simulink model "Platoon"  (Simulink 8.8)
settings: Solver=ode45  StartTime=0  StopTime=120  RelTol=1e-3  EnableMultiTasking=on
libraries: Solver_SF x5
settings Model: Creator=dhall  LastModifiedBy=mkhan  ExtModeTrigMode=oneshot  ExtModeArmWhenConnect=off
settings DataIOCC: LimitDataPoints=off  SignalLoggingName=sigsOut
settings OptimizationCC: BooleanDataType=off  LocalBlockOutputs=off  InitFltsAndDblsToZero=on
settings DebuggingCC: SaveWithParameterizedLinksMsg=none  SignalResolutionControl=TryResolveAllWithWarning  MultiTaskDSMMsg=warning  MultiTaskCondExecSysMsg=none  SFExecutionAtInitializationDiag=warning
settings HardwareCC: TargetUnknown=on
settings GRTTargetCC: TargetFcnLib=ansi_tfl_tmw.mat  CompOptLevelCompliant=off
settings ConfigComp: CovSFcnEnable=off

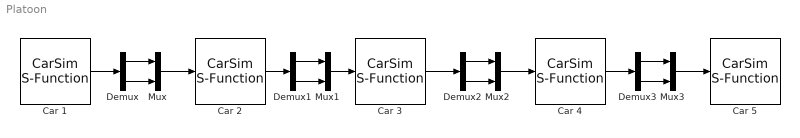
== system Platoon ==
  Car 1 : Solver_SF/CarSim S-Function  Priority=1  SIMFILE=Platoon_Car_1.sim  Run_RTs=off  vs_state_ind=Run  StopMode_ind=Vehicle Model
  Car 2 : Solver_SF/CarSim S-Function  Priority=1  SIMFILE=Platoon_Car_2.sim  Run_RTs=off  vs_state_ind=Run  StopMode_ind=Vehicle Model
  Car 3 : Solver_SF/CarSim S-Function  Priority=1  SIMFILE=Platoon_Car_3.sim  Run_RTs=off  vs_state_ind=Run  StopMode_ind=Vehicle Model
  Car 4 : Solver_SF/CarSim S-Function  Priority=1  SIMFILE=Platoon_Car_4.sim  Run_RTs=off  vs_state_ind=Run  StopMode_ind=Vehicle Model
  Car 5 : Solver_SF/CarSim S-Function  Priority=1  SIMFILE=Platoon_Car_5.sim  Run_RTs=off  vs_state_ind=Run  StopMode_ind=Vehicle Model
  Demux{,1..3} (4 alike) : Demux  Outputs=2
  Mux{,1..3} (4 alike) : Mux  Inputs=2
  wires:
  Car 1/1 -> Demux/1
  Demux/2 -> Mux/2
  Demux/1 -> Mux/1
  Mux/1 -> Car 2/1
  Car 2/1 -> Demux1/1
  Demux1/2 -> Mux1/2
  Demux1/1 -> Mux1/1
  Mux1/1 -> Car 3/1
  Demux2/2 -> Mux2/2
  Demux2/1 -> Mux2/1
  Mux2/1 -> Car 4/1
  Car 3/1 -> Demux2/1
  Demux3/2 -> Mux3/2
  Demux3/1 -> Mux3/1
  Mux3/1 -> Car 5/1
  Car 4/1 -> Demux3/1
